simulink model "quad2rotors_control"  (R2022a)
settings: Solver=ode3  StartTime=0.0  StopTime=60  FixedStep=0.01  RelTol=1e-3  EnableMultiTasking=on
values from neighbouring files (symbols this model uses):
  g = 9.8    [init.m]    (also in init_data.m)
  m = 0.18    [init.m]    (also in init_data.m)
undefined symbols (not defined in the file or in its folder): attitude_control, dThtdPhidPsi2pqr, model2rotors, position_control, pqr2dThtdPhidPsi
libraries: simulink x2
settings Model: Creator=smishra  LastModifiedBy=Giacomo Battaglia
settings SolverCC: AlgebraicLoopSolver=TrustRegion
settings DataIOCC: LimitDataPoints=on  SaveFormat=Array  ReturnWorkspaceOutputs=off  Refine=5
settings OptimizationCC: LifeSpan=inf
settings DebuggingCC: UnconnectedInputMsg=warning  UnconnectedOutputMsg=warning  UnconnectedLineMsg=warning  SFUnexpectedBacktrackingDiag=warning  SFNoUnconditionalDefaultTransitionDiag=warning  SFExecutionAtInitializationDiag=none  SFMachineParentedDataDiag=warning  ArithmeticOperatorsInVariantConditions=warning
settings HardwareCC: ProdBitPerPointer=32  ProdBitPerSizeT=32  ProdBitPerPtrDiffT=32  ProdLargestAtomicFloat=None  ProdIntDivRoundTo=Undefined  ProdEndianess=Unspecified  ProdWordSize=32  ProdHWDeviceType=32-bit Generic
settings ModelReferenceCC: PropagateSignalLabelsOutOfModel=off
settings SFSimCC: SimUseLocalCustomCode=off  CustomCodeUndefinedFunction=UseInterfaceOnly
settings RTWCC: RTWUseLocalCustomCode=off  DLArmComputeVersion=19.05
settings CodeAppCC: StateflowObjectComments=on
settings GRTTargetCC: TargetLangStandard=C89/C90 (ANSI)
settings ConfigComp: CovMetricSettings=dw  CovSaveCumulativeToWorkspaceVar=on  CovSaveSingleToWorkspaceVar=on  CovExternalEMLEnable=off

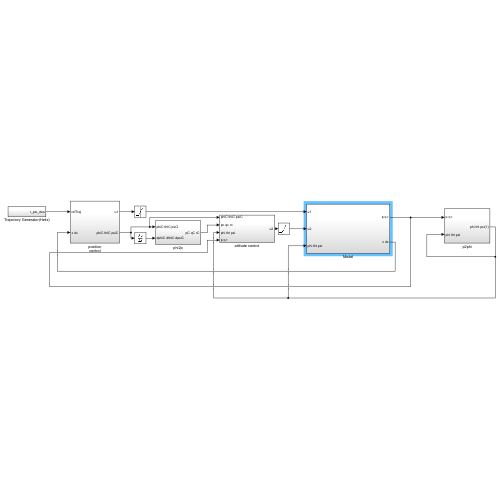
[thumbnail: Simulink's stored preview of the top-level diagram]
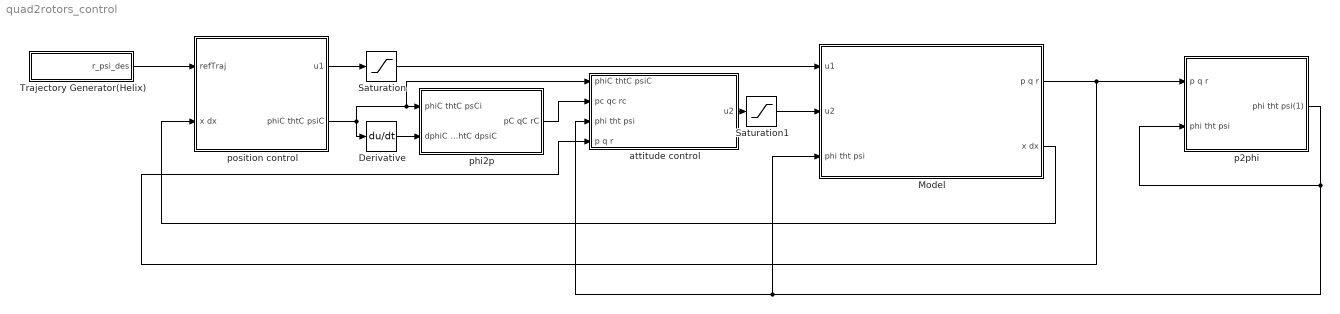
== system quad2rotors_control ==
  Derivative : Derivative
  Model : Subsystem
  Saturation : Saturate  UpperLimit=2*m*g  LowerLimit=0
  Saturation1 : Saturate  UpperLimit=0.2  LowerLimit=-0.2
  Trajectory Generator(Helix) : Subsystem
  attitude control : Subsystem
  p2phi : Subsystem
  phi2p : Subsystem
  position control : Subsystem
  wires:
  position control/2(phiC thtC psiC) -> Derivative/1, attitude control/1(phiC thtC psiC), phi2p/1(phiC thtC psCi)
  Derivative/1 -> phi2p/2(dphiC dthtC dpsiC)
  phi2p/1(pC qC rC) -> attitude control/2(pc qc rc)
  Model/2(x dx) -> position control/2(x dx)
  Model/1(p q r) -> attitude control/4(p q r), p2phi/1(p q r)
  p2phi/1(phi tht psi(1)) -> p2phi/2(phi tht psi), attitude control/3(phi tht psi), Model/3(phi tht psi)
  position control/1(u1) -> Saturation/1
  Saturation/1 -> Model/1(u1)
  attitude control/1(u2) -> Saturation1/1
  Saturation1/1 -> Model/2(u2)
  Trajectory Generator(Helix)/1(r_psi_des) -> position control/1(refTraj)

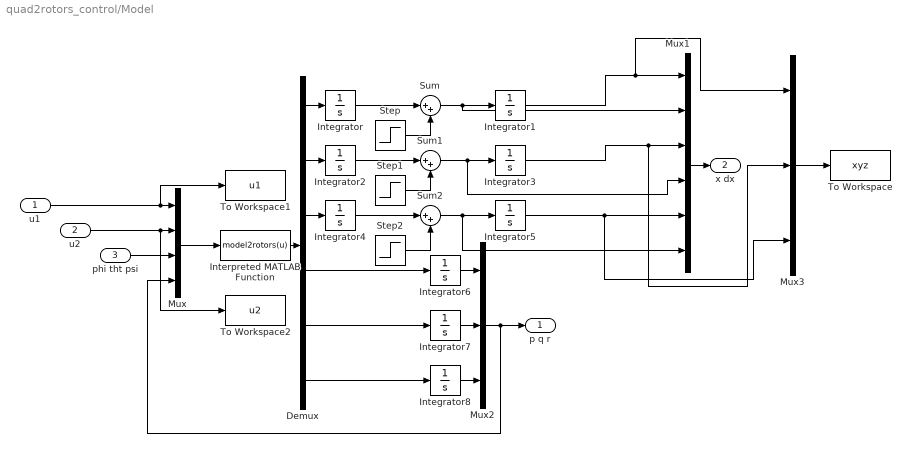
== system quad2rotors_control/Model ==
  u1 : Inport
  u2 : Inport  Port=2
  phi tht psi : Inport  Port=3
  Demux : Demux  Outputs=6
  Integrator{,1..2,4,6..8} (7 alike) : Integrator
  Integrator3 : Integrator  InitialCondition=8
  Integrator5 : Integrator  InitialCondition=-8
  Interpreted MATLAB Function : MATLABFcn  MATLABFcn=model2rotors(u)  OutputDimensions=6
  Mux : Mux
  Mux1 : Mux  Inputs=6
  Mux2 : Mux  Inputs=3
  Mux3 : Mux  Inputs=3
  Step : Step  Time=25  After=0  SampleTime=0
  Step1 : Step  Time=25  After=0  SampleTime=0
  Step2 : Step  Time=25  After=0  SampleTime=0
  Sum : Sum  Inputs=|++
  Sum1 : Sum  Inputs=|++
  Sum2 : Sum  Inputs=|++
  To Workspace : ToWorkspace  VariableName=xyz  SampleTime=-1
  To Workspace1 : ToWorkspace  VariableName=u1  SampleTime=-1
  To Workspace2 : ToWorkspace  VariableName=u2  SampleTime=-1
  p q r : Outport
  x dx : Outport  Port=2
  wires:
  Integrator5/1 -> Mux3/3, Mux1/5
  Mux2/1 -> Mux/4, p q r/1
  Mux1/1 -> x dx/1
  Mux/1 -> Interpreted MATLAB Function/1
  Integrator3/1 -> Mux3/2, Mux1/3
  Demux/3 -> Integrator4/1
  Demux/1 -> Integrator/1
  Integrator1/1 -> Mux3/1, Mux1/1
  Integrator7/1 -> Mux2/2
  Interpreted MATLAB Function/1 -> Demux/1
  Integrator8/1 -> Mux2/3
  Demux/2 -> Integrator2/1
  Integrator6/1 -> Mux2/1
  phi tht psi/1 -> Mux/3
  Mux3/1 -> To Workspace/1
  u1/1 -> To Workspace1/1, Mux/1
  u2/1 -> To Workspace2/1, Mux/2
  Demux/4 -> Integrator6/1
  Demux/5 -> Integrator7/1
  Demux/6 -> Integrator8/1
  Integrator/1 -> Sum/1
  Sum/1 -> Mux1/2, Integrator1/1
  Integrator2/1 -> Sum1/1
  Sum1/1 -> Mux1/4, Integrator3/1
  Integrator4/1 -> Sum2/1
  Sum2/1 -> Mux1/6, Integrator5/1
  Step/1 -> Sum/2
  Step1/1 -> Sum1/2
  Step2/1 -> Sum2/2

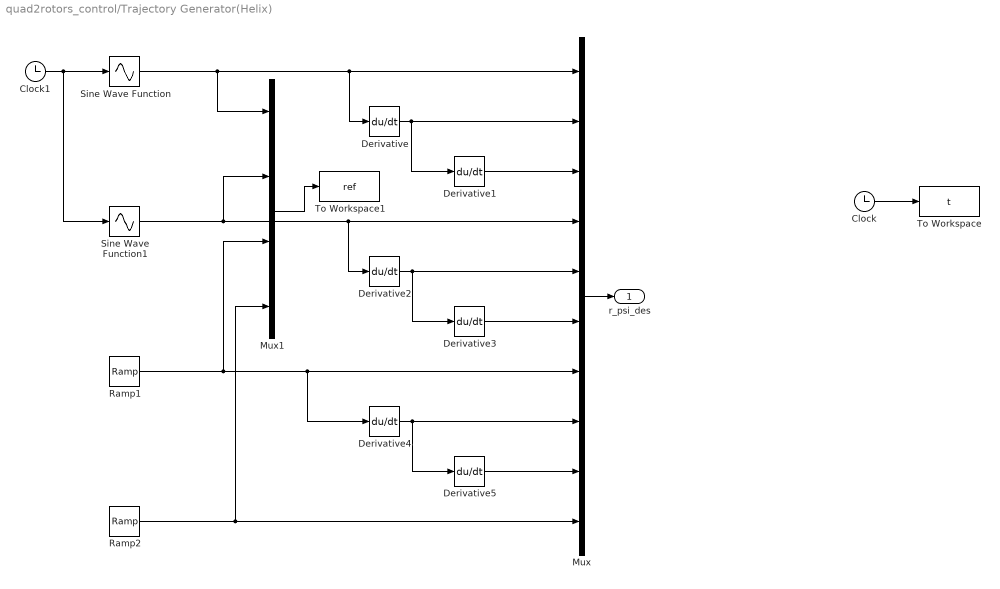
== system quad2rotors_control/Trajectory Generator(Helix) ==
  Clock : Clock
  Clock1 : Clock
  Derivative{,1..5} (6 alike) : Derivative
  Mux : Mux  Inputs=10
  Mux1 : Mux
  Ramp1 : simulink/Sources/Ramp  slope=0.2  start=0  InitialOutput=-8
  Ramp2 : simulink/Sources/Ramp  slope=0  start=0  InitialOutput=0
  Sine Wave Function : Sin  TimeSource=Use external signal  Amplitude=8  Frequency=0.1  SampleTime=0
  Sine Wave Function1 : Sin  TimeSource=Use external signal  Amplitude=8  Frequency=0.1  Phase=pi/2  SampleTime=0
  To Workspace : ToWorkspace  VariableName=t  SampleTime=-1
  To Workspace1 : ToWorkspace  VariableName=ref  SampleTime=-1
  r_psi_des : Outport
  wires:
  Derivative2/1 -> Mux/5, Derivative3/1
  Derivative4/1 -> Mux/8, Derivative5/1
  Derivative/1 -> Mux/2, Derivative1/1
  Derivative1/1 -> Mux/3
  Derivative3/1 -> Mux/6
  Derivative5/1 -> Mux/9
  Sine Wave Function/1 -> Mux1/1, Mux/1, Derivative/1
  Ramp2/1 -> Mux1/4, Mux/10
  Mux/1 -> r_psi_des/1
  Clock/1 -> To Workspace/1
  Clock1/1 -> Sine Wave Function1/1, Sine Wave Function/1
  Ramp1/1 -> Mux1/3, Derivative4/1, Mux/7
  Mux1/1 -> To Workspace1/1
  Sine Wave Function1/1 -> Mux1/2, Derivative2/1, Mux/4

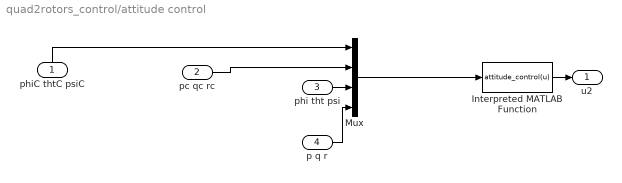
== system quad2rotors_control/attitude control ==
  phiC thtC psiC : Inport
  pc qc rc : Inport  Port=2
  phi tht psi : Inport  Port=3
  p q r : Inport  Port=4
  Interpreted MATLAB Function : MATLABFcn  MATLABFcn=attitude_control(u)  OutputDimensions=3
  Mux : Mux
  u2 : Outport
  wires:
  Mux/1 -> Interpreted MATLAB Function/1
  pc qc rc/1 -> Mux/2
  p q r/1 -> Mux/4
  phi tht psi/1 -> Mux/3
  Interpreted MATLAB Function/1 -> u2/1
  phiC thtC psiC/1 -> Mux/1

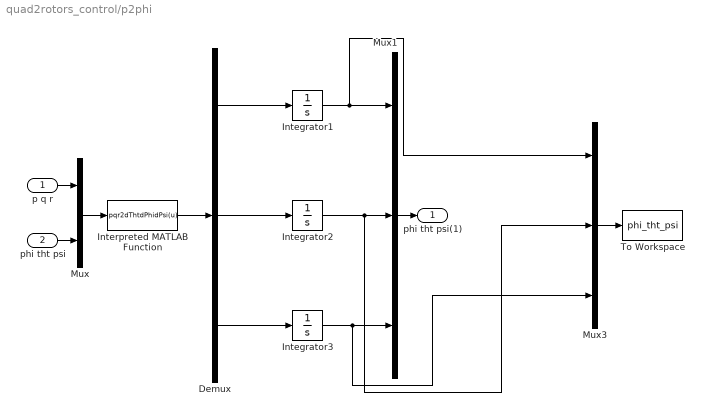
== system quad2rotors_control/p2phi ==
  p q r : Inport
  phi tht psi : Inport  Port=2
  Demux : Demux  Outputs=3
  Integrator1 : Integrator
  Integrator2 : Integrator
  Integrator3 : Integrator
  Interpreted MATLAB Function : MATLABFcn  MATLABFcn=pqr2dThtdPhidPsi(u)  OutputDimensions=3
  Mux : Mux  Inputs=2
  Mux1 : Mux  Inputs=3
  Mux3 : Mux  Inputs=3
  To Workspace : ToWorkspace  VariableName=phi_tht_psi  SampleTime=-1
  phi tht psi(1) : Outport
  wires:
  Integrator3/1 -> Mux3/3, Mux1/3
  Mux1/1 -> phi tht psi(1)/1
  Interpreted MATLAB Function/1 -> Demux/1
  Demux/3 -> Integrator3/1
  Demux/1 -> Integrator1/1
  Mux/1 -> Interpreted MATLAB Function/1
  Demux/2 -> Integrator2/1
  Integrator1/1 -> Mux3/1, Mux1/1
  phi tht psi/1 -> Mux/2
  p q r/1 -> Mux/1
  Integrator2/1 -> Mux3/2, Mux1/2
  Mux3/1 -> To Workspace/1

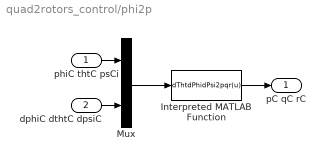
== system quad2rotors_control/phi2p ==
  phiC thtC psCi : Inport
  dphiC dthtC dpsiC : Inport  Port=2
  Interpreted MATLAB Function : MATLABFcn  MATLABFcn=dThtdPhidPsi2pqr(u)  OutputDimensions=3
  Mux : Mux  Inputs=2
  pC qC rC : Outport
  wires:
  Mux/1 -> Interpreted MATLAB Function/1
  phiC thtC psCi/1 -> Mux/1
  Interpreted MATLAB Function/1 -> pC qC rC/1
  dphiC dthtC dpsiC/1 -> Mux/2

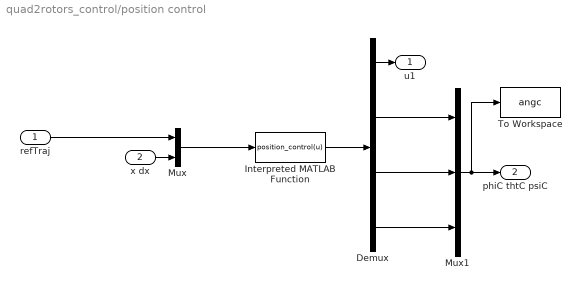
== system quad2rotors_control/position control ==
  refTraj : Inport
  x dx : Inport  Port=2
  Demux : Demux
  Interpreted MATLAB Function : MATLABFcn  MATLABFcn=position_control(u)  OutputDimensions=4
  Mux : Mux  Inputs=2
  Mux1 : Mux  Inputs=3
  To Workspace : ToWorkspace  VariableName=angc  SampleTime=-1
  u1 : Outport
  phiC thtC psiC : Outport  Port=2
  wires:
  Interpreted MATLAB Function/1 -> Demux/1
  Mux/1 -> Interpreted MATLAB Function/1
  refTraj/1 -> Mux/1
  Demux/4 -> Mux1/3
  x dx/1 -> Mux/2
  Demux/2 -> Mux1/1
  Demux/1 -> u1/1
  Demux/3 -> Mux1/2
  Mux1/1 -> To Workspace/1, phiC thtC psiC/1
